simulink model "battery_project"  (R2023b)
settings: Solver=VariableStepAuto  StartTime=0.0  StopTime=600  RelTol=1e-3
model workspace (MAT data in the model file):
  A = Simulink.Parameter
  A.DataType = 'auto'
  A.Complexity = 'real'
  A.Dimensions = [0 0]
  B = 1
  C = 1
  D = 1
values from neighbouring files (symbols this model uses):
  A_mat = [0, 0; 0, - 1 / (C*R1)]    [state_space_1_vars.m]
  B_mat = [1/Q; 1/C]    [state_space_1_vars.m]
  C_dummy = eye(2)    [state_space_1_vars.m]
  D_dummy = [0;0]    [state_space_1_vars.m]
  p_0 = 3.28229043218463    (= 3.28229043218)    [state_space_1_vars.m]
  p_1 = 3.74878321288425    (= 3.74878321288)    [state_space_1_vars.m]
  p_2 = -19.7495647885364    (= -19.7495647885)    [state_space_1_vars.m]
  p_3 = 48.7434451832868    (= 48.7434451833)    [state_space_1_vars.m]
  p_4 = -52.9516197704481    (= -52.9516197704)    [state_space_1_vars.m]
  p_5 = 20.9865358625928    (= 20.9865358626)    [state_space_1_vars.m]
  x0 = [z0, V_c0]    [state_space_1_vars.m]
settings Model: Creator=Teama  LastModifiedBy=Teama
settings OptimizationCC: ReuseModelBlockBuffer=off

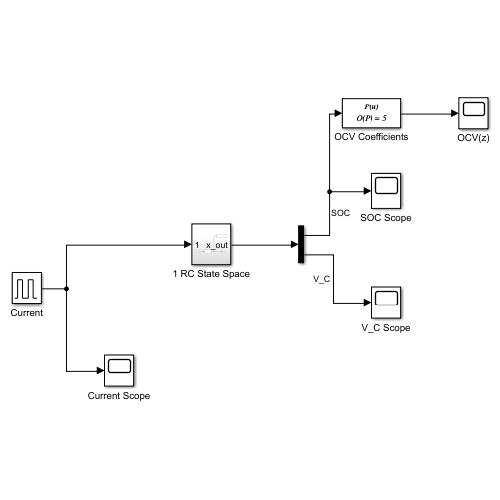
[thumbnail: Simulink's stored preview of the top-level diagram]
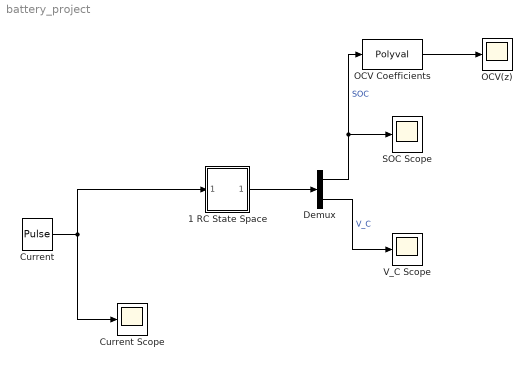
== system battery_project ==
  1 RC State Space : Subsystem
  Current : DiscretePulseGenerator  PulseType=Time based  Amplitude=-5  Period=40  PulseWidth=50
  Current Scope : Scope
  Demux : Demux  Outputs=2
  OCV Coefficients : Polyval  Coefs=[p_5,p_4,p_3, p_2, p_1, p_0]
  OCV(z) : Scope
  SOC Scope : Scope
  V_C Scope : Scope
  wires:
  Current/1 -> 1 RC State Space/1(In1), Current Scope/1
  1 RC State Space/1(x_out) -> Demux/1
  Demux/1 -> OCV Coefficients/1, SOC Scope/1  "SOC"
  Demux/2 -> V_C Scope/1  "V_C"
  OCV Coefficients/1 -> OCV(z)/1

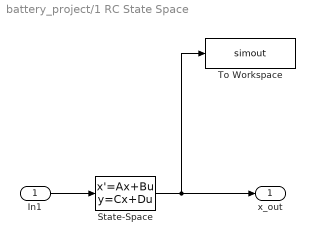
== system battery_project/1 RC State Space ==
  In1 : Inport
  State-Space : StateSpace  A=A_mat  B=B_mat  C=C_dummy  D=D_dummy  InitialCondition=x0
  To Workspace : ToWorkspace  VariableName=simout  SaveFormat=Timeseries  SampleTime=-1
  x_out : Outport
  wires:
  State-Space/1 -> x_out/1, To Workspace/1
  In1/1 -> State-Space/1
